simulink model "Representacion"  (R2023b)
settings: Solver=VariableStepAuto  StartTime=0.0  StopTime=20  RelTol=1e-3
InitFcn:
  | Ip = 0.0079; % kg*m^2
  | Mc = 0.7031; % kg
  | lp = 0.3302; % m
  | Mp = 0.23; % kg
  | Fe = 0; % N
  | Beq = 4.3; % Ns/m
  | g = 9.81; % m/s^2
  | Bp = 0.0024; % Nms/rad
settings Model: Creator=adria  LastModifiedBy=adria

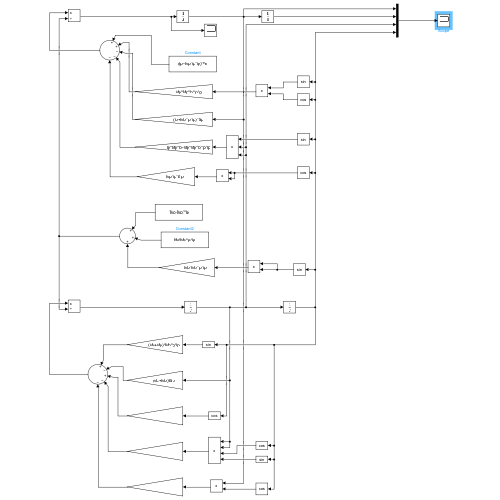
[thumbnail: Simulink's stored preview of the top-level diagram]
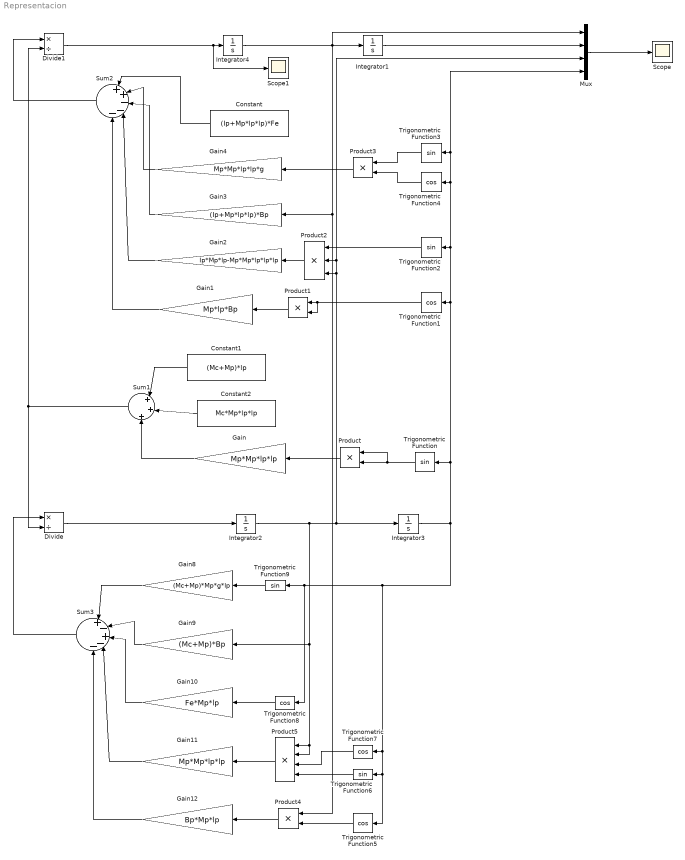
== system Representacion ==
  Constant : Constant  Value=(Ip+Mp*lp*lp)*Fe
  Constant1 : Constant  Value=(Mc+Mp)*lp
  Constant2 : Constant  Value=Mc*Mp*lp*lp
  Divide : Product  Inputs=*/
  Divide1 : Product  Inputs=*/
  Gain : Gain  Gain=Mp*Mp*lp*lp
  Gain1 : Gain  Gain=Mp*lp*Bp
  Gain10 : Gain  Gain=Fe*Mp*lp
  Gain11 : Gain  Gain=Mp*Mp*lp*lp
  Gain12 : Gain  Gain=Bp*Mp*lp
  Gain2 : Gain  Gain=Ip*Mp*lp-Mp*Mp*lp*lp*lp
  Gain3 : Gain  Gain=(Ip+Mp*lp*lp)*Bp
  Gain4 : Gain  Gain=Mp*Mp*lp*lp*g
  Gain8 : Gain  Gain=(Mc+Mp)*Mp*g*lp
  Gain9 : Gain  Gain=(Mc+Mp)*Bp
  Integrator1 : Integrator
  Integrator2 : Integrator
  Integrator3 : Integrator  InitialCondition=3.14/180
  Integrator4 : Integrator  UpperSaturationLimit=100  LowerSaturationLimit=-100
  Mux : Mux
  Product{,1,3..4} (4 alike) : Product
  Product2 : Product  Inputs=3
  Product5 : Product  Inputs=4
  Scope : Scope
  Scope1 : Scope
  Sum1 : Sum  Inputs=|+|+|+
  Sum2 : Sum  Inputs=|+|+|-|-|-
  Sum3 : Sum  Inputs=|+|-|+|-|-
  Trigonometric Function{,2..3,6,9} (5 alike) : Trigonometry
  Trigonometric Function{1,4..5,7..8} (5 alike) : Trigonometry  Operator=cos
  wires:
  Integrator4/1 -> Product4/1, Gain3/1, Integrator1/1, Mux/1
  Integrator1/1 -> Mux/2
  Trigonometric Function9/1 -> Gain8/1
  Gain9/1 -> Sum3/2
  Integrator3/1 -> Trigonometric Function5/1, Trigonometric Function6/1, Trigonometric Function7/1, Trigonometric Function8/1, Trigonometric Function9/1, Mux/4, Trigonometric Function3/1, Trigonometric Function4/1, Trigonometric Function2/1, Trigonometric Function1/1, Trigonometric Function/1
  Mux/1 -> Scope/1
  Trigonometric Function8/1 -> Gain10/1
  Trigonometric Function6/1 -> Product5/4
  Gain2/1 -> Sum2/4
  Gain3/1 -> Sum2/3
  Product5/1 -> Gain11/1
  Integrator2/1 -> Gain9/1, Product5/2, Product5/1, Product2/2, Mux/3, Product2/3, Integrator3/1
  Product4/1 -> Gain12/1
  Constant1/1 -> Sum1/1
  Gain10/1 -> Sum3/3
  Gain8/1 -> Sum3/1
  Gain1/1 -> Sum2/5
  Product1/1 -> Gain1/1
  Trigonometric Function7/1 -> Product5/3
  Gain4/1 -> Sum2/2
  Gain12/1 -> Sum3/5
  Sum3/1 -> Divide/1
  Trigonometric Function3/1 -> Product3/1
  Trigonometric Function2/1 -> Product2/1
  Divide/1 -> Integrator2/1
  Product/1 -> Gain/1
  Trigonometric Function4/1 -> Product3/2
  Trigonometric Function/1 -> Product/2, Product/1
  Product2/1 -> Gain2/1
  Trigonometric Function1/1 -> Product1/2, Product1/1
  Product3/1 -> Gain4/1
  Gain/1 -> Sum1/3
  Sum1/1 -> Divide1/2, Divide/2
  Constant2/1 -> Sum1/2
  Trigonometric Function5/1 -> Product4/2
  Divide1/1 -> Scope1/1, Integrator4/1
  Sum2/1 -> Divide1/1
  Gain11/1 -> Sum3/4
  Constant/1 -> Sum2/1
